simulink model "model"  (R2020b)
settings: Solver=VariableStepAuto  StartTime=0.0  StopTime=10.0  RelTol=1e-3
settings Model: Creator=SAGAR  LastModifiedBy=SAGAR

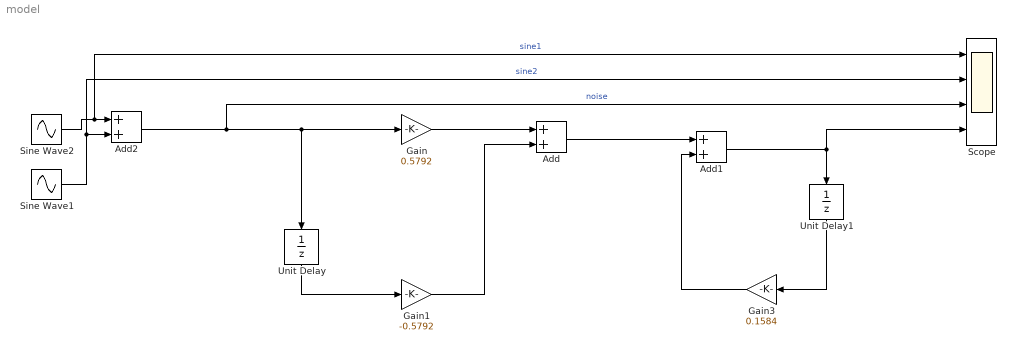
== system model ==
  Add : Sum
  Add1 : Sum
  Add2 : Sum
  Gain : Gain  Gain=0.5792
  Gain1 : Gain  Gain=-0.5792
  Gain3 : Gain  Gain=0.1584
  Scope : Scope  NumInputPorts=4
  Sine Wave1 : Sin  Frequency=62840  SampleTime=0
  Sine Wave2 : Sin  SampleTime=0
  Unit Delay : UnitDelay  SampleTime=-1  HasFrameUpgradeWarning=on
  Unit Delay1 : UnitDelay  SampleTime=-1  HasFrameUpgradeWarning=on
  wires:
  Gain/1 -> Add/1
  Add2/1 -> Scope/3, Unit Delay/1, Gain/1  "noise"
  Unit Delay/1 -> Gain1/1
  Gain1/1 -> Add/2
  Add/1 -> Add1/1
  Gain3/1 -> Add1/2
  Add1/1 -> Scope/4, Unit Delay1/1
  Unit Delay1/1 -> Gain3/1
  Sine Wave2/1 -> Scope/1, Add2/1  "sine1"
  Sine Wave1/1 -> Scope/2, Add2/2  "sine2"
